simulink model "ukf_cfg2"  (Simulink 9.2)
settings: Solver=FixedStepDiscrete  StartTime=0.0  StopTime=5  FixedStep=0.05  RelTol=1e-3  EnableMultiTasking=on
InitFcn:
  | R = 0.2; % Variance of the measurement noise v[k]
  | 
  | ukf.ProcessNoise = diag([0.02 0.1]);
  | 
  | T = 0.05; % [s] Filter sample time
  | timeVector = 0:T:5;
  | [~,xTrue]=ode45(@vdp1,timeVector,[2;0]);
  | 
  | rng(1); % Fix the random number generator for reproducible results
  | yTrue = xTrue(:,1);
  | yMeas = yTrue .* (1+sqrt(R)*randn(size(yTrue))); % sqrt(R): Standard deviation of noise
  | 
  | yMeasSim = [timeVector',yMeas(:,1)];
libraries: sharedTrackingLibrary x1
settings Model: Creator=igeorgie  LastModifiedBy=GEI1SF4  PauseTimes=93.4  SnapshotBufferSize=5  SnapshotInterval=5
settings SolverCC: AutoInsertRateTranBlk=on
settings DataIOCC: SignalLoggingSaveFormat=Dataset
settings DebuggingCC: SolverPrmCheckMsg=warning  FcnCallInpInsideContextMsg=error  StateNameClashWarn=none
settings GRTTargetCC: CombineOutputUpdateFcns=on  GRTInterface=off

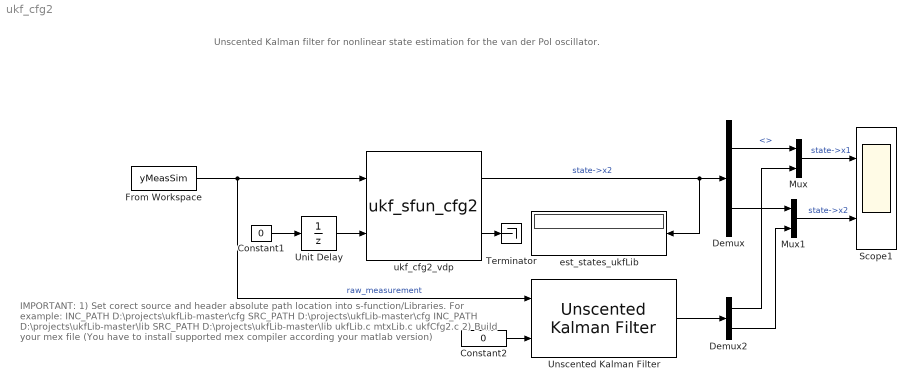
== system ukf_cfg2 ==
  note: Unscented Kalman filter for nonlinear state estimation for the van der Pol oscillator.
  note: IMPORTANT:
      | 1) Set corect source and header absolute path location into s-function/Libraries. For example:
      | INC_PATH D:\projects\ukfLib-master\cfg
      | SRC_PATH D:\projects\ukfLib-master\cfg
      | INC_PATH D:\projects\ukfLib-master\lib
      | SRC_PATH D:\projects\ukfLib-master\lib
      | ukfLib.c
      | mtxLib.c
      | ukfCfg2.c
      | 2) Build your mex file (You have to install supported mex compiler according your matlab version)
  Constant1 : Constant  Value=0  OutDataTypeStr=double  SampleTime=0.1
  Constant2 : Constant  Value=0  OutDataTypeStr=double  SampleTime=0.05
  Demux : Demux  Outputs=2
  Demux2 : Demux  Outputs=2
  From Workspace : FromWorkspace  VariableName=yMeasSim  SampleTime=0.05  OutputAfterFinalValue=Holding final value
  Mux : Mux  Inputs=2
  Mux1 : Mux  Inputs=2
  Scope1 : Scope  NumInputPorts=2
  Terminator : Terminator
  Unit Delay : UnitDelay  InitialCondition=1  SampleTime=0.05
  Unscented Kalman Filter : sharedTrackingLibrary/Unscented Kalman Filter  StateTransitionFcn=vdpStateFcn  HasAdditiveProcessNoise=Additive  ProcessNoise=[0.02,0;0,0.1]  HasTimeVaryingProcessNoise=off  HasStateTransitionFcnExtraArgument=0  InitialState=[2 0]  InitialStateCovariance=[1,0,;0,1]  Alpha=0.1  Beta=2  Kappa=0  MeasurementFcn1=vdpMeasurementNonAdditiveNoiseFcn  HasMeasurementEnablePort1=off  HasAdditiveMeasurementNoise1=Additive  MeasurementNoise1=0.2  HasTimeVaryingMeasurementNoise1=off  HasMeasurementFcnExtraArgument1=1  MeasurementFcn2=myMeasurementFcn  HasMeasurementEnablePort2=off  HasAdditiveMeasurementNoise2=Additive  MeasurementNoise2=1  HasTimeVaryingMeasurementNoise2=off  HasMeasurementFcnExtraArgument2=0  MeasurementFcn3=myMeasurementFcn  HasMeasurementEnablePort3=off  HasAdditiveMeasurementNoise3=Additive  MeasurementNoise3=1  HasTimeVaryingMeasurementNoise3=off  HasMeasurementFcnExtraArgument3=0  MeasurementFcn4=myMeasurementFcn  HasMeasurementEnablePort4=off  HasAdditiveMeasurementNoise4=Additive  MeasurementNoise4=1  HasTimeVaryingMeasurementNoise4=off  HasMeasurementFcnExtraArgument4=0  MeasurementFcn5=myMeasurementFcn  HasMeasurementEnablePort5=off  HasAdditiveMeasurementNoise5=Additive  MeasurementNoise5=1  HasTimeVaryingMeasurementNoise5=off  HasMeasurementFcnExtraArgument5=0  EnableMultirate=off  StateTransitionFcnSampleTime=1  MeasurementFcn1SampleTime=1  MeasurementFcn2SampleTime=1  MeasurementFcn3SampleTime=1  MeasurementFcn4SampleTime=1  MeasurementFcn5SampleTime=1  UseCurrentEstimator=on  OutputStateCovariance=off  DataType=double  SampleTime=0.05  NumberOfMeasurements=1
      settings: SourceProductName=Control System Toolbox  SourceProductBaseCode=CT
  est_states_ukfLib : Display
  ukf_cfg2_vdp : S-Function  InitFcn=try, set_param(gcb,'FunctionName','ukf_sfun_cfg2'), end  FunctionName=ukf_sfun_cfg2  SFunctionModules=ukf_sfun_cfg2_wrapper ukfLib mtxLib ukfCfg2  WizardData=DataTag0  SFunctionDeploymentMode=off  EnableBusSupport=off  mask(S-Function Builder){}
      mask help: Simulink:masks:SFunctionBuilder_MD
      mask init:
      | val = [[.9  0.75 0.75 1 1 .9 .9 1]',[1 1 0.75 0.75 .9 .9 1 .9]'];try , sys = get_param(gcb,'SfunBuilderFcnName');if isempty(sys), sys = get_param(gcb,'FunctionName'); end,catch, sys = get_param(gcb,'FunctionName'); end
      settings: CopyFcn=set_param(gcbh,'LinkStatus','none')  PreSaveFcn=try, set_param(gcb,'FunctionName','ukf_sfun_cfg2'), end  OpenFcn=sfunctionwizard(gcbh)
      mask Display:
      | plot(val(:,1),val(:,2))
      | disp(sys)
      | port_label('input',1,'meas')
      | port_label('input',2,'Init')
      | port_label('output',1,'states')
      | port_label('output',2,'y_mean')
  wires:
  Unit Delay/1 -> ukf_cfg2_vdp/2
  Constant1/1 -> Unit Delay/1
  Demux/1 -> Mux/1  "<>"
  Demux/2 -> Mux1/1
  Mux/1 -> Scope1/1  "state->x1"
  Mux1/1 -> Scope1/2  "state->x2"
  ukf_cfg2_vdp/2 -> Terminator/1
  ukf_cfg2_vdp/1 -> est_states_ukfLib/1, Demux/1  "state->x2"
  From Workspace/1 -> Unscented Kalman Filter/1, ukf_cfg2_vdp/1  "raw_measurement"
  Constant2/1 -> Unscented Kalman Filter/2
  Unscented Kalman Filter/1 -> Demux2/1
  Demux2/1 -> Mux/2
  Demux2/2 -> Mux1/2
